simulink model "nbus_dyna_angle_change"  (R2023a)
settings: Solver=ode23  StartTime=0.0  StopTime=10  FixedStep=0.01  RelTol=1e-3
values from neighbouring files (symbols this model uses):
  Load = 1.4062    [ee5802.m]
  rpu = R/Rbase    [ee5802.m]
settings Model: Creator=XPS  LastModifiedBy=Jecordjo

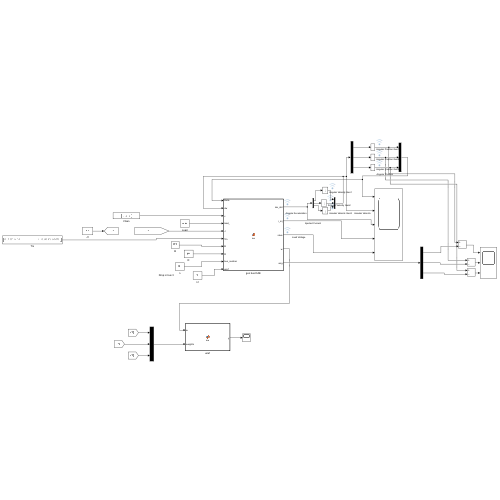
[thumbnail: Simulink's stored preview of the top-level diagram]
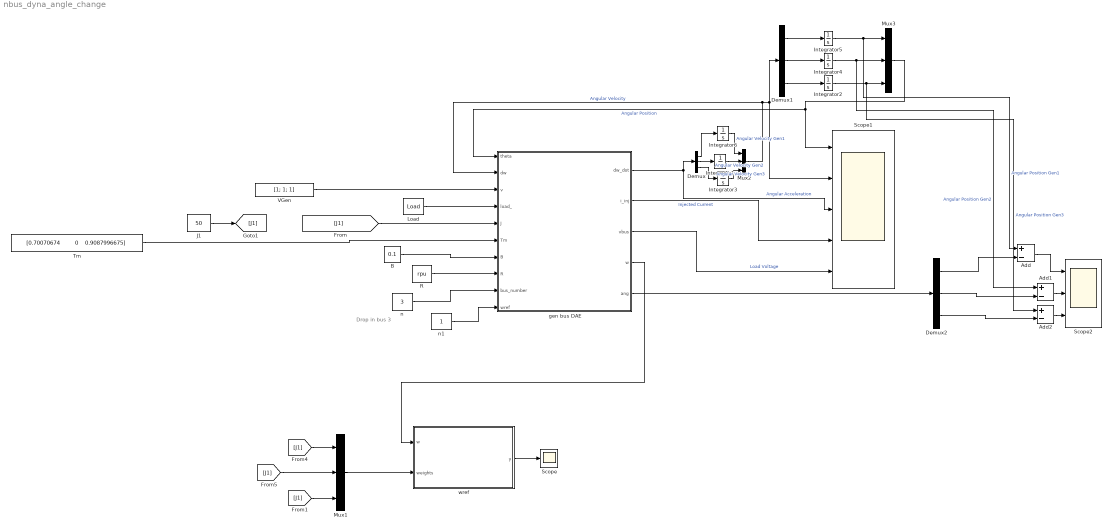
== system nbus_dyna_angle_change ==
  note: Drop in bus 3
  Add : Sum  Inputs=+-
  Add1 : Sum  Inputs=+-
  Add2 : Sum  Inputs=+-
  B : Constant  Value=0.1
  Demux : Demux  Outputs=3
  Demux1 : Demux  Outputs=3
  Demux2 : Demux  Outputs=3
  Integrator{1,3,5..6} (4 alike) : Integrator
  Integrator2 : Integrator  InitialCondition=0.1019
  Integrator4 : Integrator  InitialCondition=0.22339030558521
  J1 : Constant  Value=50
  Load : Constant  Value=Load
  Mux1 : Mux  Inputs=3
  Mux2 : Mux  Inputs=3
  Mux3 : Mux  Inputs=3
  R : Constant  Value=rpu
  Scope : Scope
  Scope1 : Scope  NumInputPorts=5
  Scope2 : Scope  NumInputPorts=3
  Tm : Constant  Value="[0.70070674         0    0.9087996675]"
  VGen : Constant  Value=[1; 1; 1]
  gen bus DAE : MATLAB Function  TreatAsAtomicUnit=on
  n : Constant  Value=3
  n1 : Constant
  wref : MATLAB Function  TreatAsAtomicUnit=on
  wires:
  gen bus DAE/1(dw_dot) -> Scope1/3, Demux/1  "Angular Acceleration"
  Mux2/1 -> gen bus DAE/2(dw), Scope1/2, Demux1/1  "Angular Velocity"
  J1/1 -> [J1]
  gen bus DAE/2(i_inj) -> Scope1/4  "Injected Current"
  B/1 -> gen bus DAE/7(B)
  VGen/1 -> gen bus DAE/3(v)
  gen bus DAE/3(vbus) -> Scope1/5  "Load Voltage"
  Tm/1 -> gen bus DAE/6(Tm)
  n/1 -> gen bus DAE/9(bus_number)
  R/1 -> gen bus DAE/8(R)
  Load/1 -> gen bus DAE/4(load_)
  Mux3/1 -> Scope1/1, gen bus DAE/1(theta)  "Angular Position"
  n1/1 -> gen bus DAE/10(wref)
  [J1] -> gen bus DAE/5(J)
  gen bus DAE/4(w) -> wref/1(w)
  Mux1/1 -> wref/2(weights)
  [J1] -> Mux1/1
  [J1] -> Mux1/2
  Demux/2 -> Integrator1/1
  Demux/3 -> Integrator3/1
  Integrator1/1 -> Mux2/2  "Angular Velocity Gen2"
  Integrator3/1 -> Mux2/3  "Angular Velocity Gen3"
  Demux1/2 -> Integrator4/1
  Demux1/3 -> Integrator2/1
  Integrator2/1 -> Add2/1, Mux3/3  "Angular Position Gen3"
  Integrator4/1 -> Add1/1, Mux3/2  "Angular Position Gen2"
  wref/1(y) -> Scope/1
  [J1] -> Mux1/3
  Integrator5/1 -> Add/1, Mux3/1  "Angular Position Gen1"
  Demux1/1 -> Integrator5/1
  Demux/1 -> Integrator6/1
  Integrator6/1 -> Mux2/1  "Angular Velocity Gen1"
  gen bus DAE/5(ang) -> Demux2/1
  Demux2/1 -> Add/2
  Demux2/2 -> Add1/2
  Demux2/3 -> Add2/2
  Add/1 -> Scope2/1
  Add1/1 -> Scope2/2
  Add2/1 -> Scope2/3

== matlab function nbus_dyna_angle_change/gen bus DAE ==
  data: theta input size=3; dw_dot output size=3; dw input; i_inj output size=3; v input size=3; load_ input; J input; Tm input; B input; vbus output; R input; bus_number input; wref input; w output; ang output
function [dw_dot, i_inj , vbus, w, ang] = fcn(theta,dw,v,load_,J,Tm,B,R,bus_number,wref)
n=bus_number;
% x0 = zeros(2,n);
w=zeros(3,1);
dw_dot = zeros(3,1);
ang=[0 0 0];
% x0(2,1) = load_(1);
% for j = 2:n
%     x0(1,j) = v(1);
%     x0(2,j) = load_(j);
% end
w=dw+[wref;wref;wref];
x0 = [v(1) v(2) v(3);1.05 0 1.01;theta(1) theta(2) theta(3)];
sol = fsolve(@(x) solving_systems_nbus(x, [v(1) v(2) v(3)], [-1 0 -1], load_, R, n, [theta(1) -1 theta(3)]),x0,optimoptions('fsolve','Display','off','Algorithm','levenberg-marquardt'));

i_inj = sol(2,:)';

vbus = sol(1,:);

ang = sol(3,:);

dw_dot(1) = (1/J)*(Tm(1) - ((v(1)*i_inj(1)*cos(sol(3,1)))/w(1)) - B*w(1) - 0.001*dw(1));
dw_dot(2) = 0;
dw_dot(3) =  (1/J)*(Tm(3) - ((v(3)*i_inj(3)*cos(sol(3,3)))/w(3)) - B*w(3) - 0.001*dw(3));

== matlab function nbus_dyna_angle_change/wref ==
  data: w input; y output; weights input
function y = fcn(w,weights)
    
y = sum(w.*(weights/sum(weights)));
